simulink model "gyro_model"  (R2021a)
settings: Solver=VariableStepAuto  StartTime=0.0  StopTime=180  FixedStep=1/95  RelTol=1e-3
values from neighbouring files (symbols this model uses):
  bias_sigma = 0.003    [gyro_params.m]
  K_misalign = 1 + epsilon    (= 1.0035)    [gyro_params.m]
  static_bias = -0.6851    [gyro_params.m]
  w = 2*pi*12.5    (= 78.5398163397)    [gyro_params.m]
  wn = 1000*2*pi    (= 6283.18530718)    [gyro_params.m]
  z = 0.707    [gyro_params.m]
  zeta = 0.707    [gyro_params.m]
undefined symbols (not defined in the file or in its folder): DiscIntNeverNeededParam
libraries: simulink x1
settings Model: Creator=abdelrahman  LastModifiedBy=abdelrahman

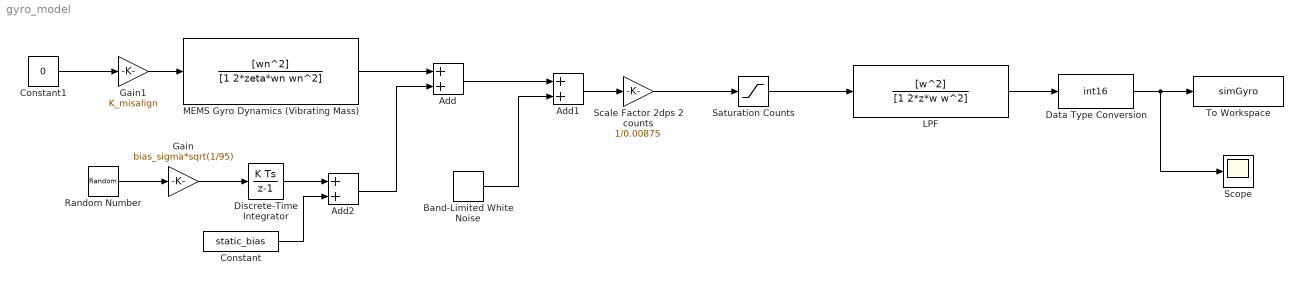
== system gyro_model ==
  Add : Sum
  Add1 : Sum
  Add2 : Sum
  Band-Limited White Noise : simulink/Sources/Band-Limited White Noise  Cov=[0.03^2]  Ts=0.1  seed=[23341]
  Constant : Constant  Value=static_bias
  Constant1 : Constant  Value=0
  Data Type Conversion : DataTypeConversion  OutMin=[-32767]  OutMax=[32767]  OutDataTypeStr=int16
  Discrete-Time Integrator : DiscreteIntegrator  SampleTime=-1  ICPrevOutput=DiscIntNeverNeededParam  ICPrevScaledInput=DiscIntNeverNeededParam
  Gain : Gain  Gain=bias_sigma*sqrt(1/95)
  Gain1 : Gain  Gain=K_misalign
  LPF : TransferFcn  Numerator=[w^2]  Denominator=[1 2*z*w w^2]
  MEMS Gyro Dynamics (Vibrating Mass) : TransferFcn  Numerator=[wn^2]  Denominator=[1 2*zeta*wn wn^2]
  Random Number : RandomNumber  SampleTime=0.1
  Saturation Counts : Saturate  UpperLimit=2^15  LowerLimit=-2^15
  Scale Factor 2dps 2 counts : Gain  Gain=1/0.00875
  Scope : Scope
  To Workspace : ToWorkspace  VariableName=simGyro  SampleTime=-1
  wires:
  Constant1/1 -> Gain1/1
  MEMS Gyro Dynamics (Vibrating Mass)/1 -> Add/1
  Add/1 -> Add1/1
  Band-Limited White Noise/1 -> Add1/2
  Add1/1 -> Scale Factor 2dps 2 counts/1
  Scale Factor 2dps 2 counts/1 -> Saturation Counts/1
  Saturation Counts/1 -> LPF/1
  LPF/1 -> Data Type Conversion/1
  Data Type Conversion/1 -> Scope/1, To Workspace/1
  Random Number/1 -> Gain/1
  Gain/1 -> Discrete-Time Integrator/1
  Discrete-Time Integrator/1 -> Add2/1
  Constant/1 -> Add2/2
  Add2/1 -> Add/2
  Gain1/1 -> MEMS Gyro Dynamics (Vibrating Mass)/1
